simulink model "Double_current_Vin_Iout_integrator_method"  (R2024a)
settings: Solver=VariableStepAuto  StartTime=0.0  StopTime=10.0  RelTol=1e-3
values from neighbouring files (symbols this model uses):
  c1 = 20    [Double_current_parameters.mat]
  c2 = 50    [Double_current_parameters.mat]
  r1 = 200    [Double_current_parameters.mat]
  r2 = 1    [Double_current_parameters.mat]
settings Model: Creator=nassa  LastModifiedBy=nassa

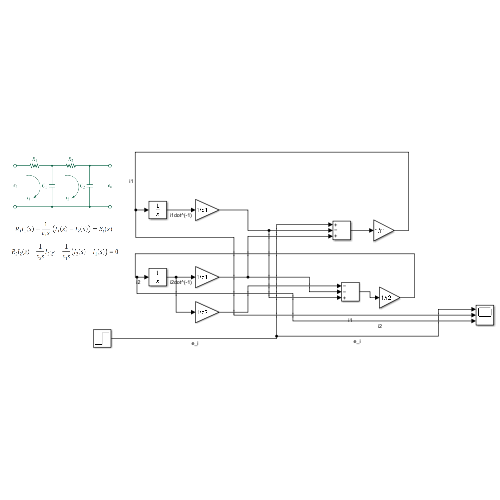
[thumbnail: Simulink's stored preview of the top-level diagram]
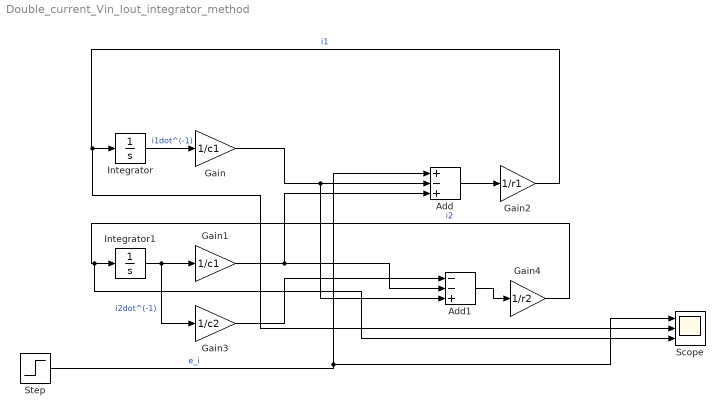
== system Double_current_Vin_Iout_integrator_method ==
  Add : Sum  Inputs=+-+
  Add1 : Sum  Inputs=--+
  Gain : Gain  Gain=1/c1
  Gain1 : Gain  Gain=1/c1
  Gain2 : Gain  Gain=1/r1
  Gain3 : Gain  Gain=1/c2
  Gain4 : Gain  Gain=1/r2
  Integrator : Integrator
  Integrator1 : Integrator
  Scope : Scope  NumInputPorts=3
  Step : Step  SampleTime=0
  wires:
  Gain2/1 -> Scope/2, Integrator/1  "i1"
  Integrator/1 -> Gain/1  "i1dot^(-1)"
  Gain4/1 -> Scope/3, Integrator1/1  "i2"
  Integrator1/1 -> Gain3/1, Gain1/1  "i2dot^(-1)"
  Step/1 -> Scope/1, Add/1  "e_i"
  Gain/1 -> Add1/3, Add/2
  Gain1/1 -> Add1/2, Add/3
  Add/1 -> Gain2/1
  Gain3/1 -> Add1/1
  Add1/1 -> Gain4/1
